simulink model "Cruise_MPC_Adaptive"  (R2018a)
settings: Solver=VariableStepAuto  StartTime=0.0  StopTime=inf  FixedStep=0.01  RelTol=1e-3  EnableMultiTasking=on
PreLoadFcn:
  | sampleTime = 0.05;
  | 
  | % Vehicle Parameters
  | R = 0.1;
  | L = 0.5;
undefined symbols (not defined in the file): C1, C2, cBW, d, Discrete, dw, I, Iw, md, Time, Waypoint
libraries: mobileRoboticsLib x2, cstblocks x2, mpclib x1, ctrlSharedLib x1, dspsrcs4 x1
settings Model: SimulationMode=accelerator  EnablePacing=on  Creator=scastro  LastModifiedBy=shravan
settings DataIOCC: LimitDataPoints=on
settings OptimizationCC: EfficientMapNaN2IntZero=off  LifeSpan=inf
settings DebuggingCC: AllowSymbolicDim=off  SFUnexpectedBacktrackingDiag=warning  SFNoUnconditionalDefaultTransitionDiag=warning  SFExecutionAtInitializationDiag=none
settings HardwareCC: TargetBitPerLong=64  TargetBitPerPointer=64  TargetBitPerSizeT=64  TargetBitPerPtrDiffT=64  TargetLongLongMode=on  TargetIntDivRoundTo=Zero  TargetEndianess=LittleEndian  TargetWordSize=64  TargetHWDeviceType=MATLAB Host  ProdEqTarget=off
settings CodeAppCC: MaxIdLength=128
settings GRTTargetCC: TargetLangStandard=C89/C90 (ANSI)  CombineOutputUpdateFcns=off  GRTInterface=on
settings ConfigComp: CovMetricSettings=dw  CovHtmlReporting=on  CovSaveCumulativeToWorkspaceVar=on  CovSaveSingleToWorkspaceVar=on  CovExternalEMLEnable=off  CovSFcnEnable=off
settings SimscapeCC: SimscapeNominalValues="[{\"value\":\"10\",\"unit\":\"V\"},{\"value\":\"1\",\"unit\":\"A\"},{\"value\":\"10\",\"unit\":\"N*m\"},{\"value\":\"10\",\"unit\":\"bar\"},{\"value\":\"100\",\"unit\":\"kJ/kg\"},{\"value\":\"1\",\"unit\":\"kW\"},{\"value\":\"300\",\"unit\":\"K\"},{\"value\":\"100\",\"unit\":\"cm^3/s\"},{\"value\":\"1\",\"unit\":\"kN\"},{\"value\":\"1\",\"unit\":\"g/cm^3\"},{\"value\":\"1\",\"unit\":\"l\"},{\"value\":\"1\",\"unit\":\"cm^2\"},{\"value\":\"60\",\"unit\":\"Hz\"}]"  SimscapeLogType=all  SimscapeLogDataHistory=10000
settings ConfigurationSet: Description=SimMechanics 2G
settings ExplorerConfigSet: InternalSimMechanicsExplorerSettings="<ExplorerConfiguration><canonicalview>default</canonicalview><AnimationSetting><BasePlaybackSpeed>1.0</BasePlaybackSpeed><PlaybackSpeedFactor>1.0</PlaybackSpeedFactor></AnimationSetting><TilePanel><TileInfo><Tiles Columns=\"1\" Count=\"1\" Rows=\"1\"><Column Weight=\"1\"/><Row Weight=\"1\"/><Tile Height=\"1\" Width=\"1\" X=\"0\" Y=\"0\"/></Tiles></TileInfo><SceneInfo><SceneViewer><BGColor><R>0.60000002384185791</R><G>0.60000002384185791</G><B>0.60000002384185791</B></BGColor><Camera><DoPerspective>off</DoPerspective><Position><X>-1.70656042355848525</X><Y>-0.974920623359631922</Y><Z>4.72930454537082046</Z></Position><Center><X>0.552860638431633689</X><Y>1.42025063411503494</Y><Z>1.4843509506914252</Z></Center><Up><X>0.664249622453917166</X><Y>0.300615402055903091</Y><Z>0.684399604848363485</Z></Up><ViewLimDist>1</ViewLimDist><YLim>2.77881717169207398</YLim><XLim>3.55928742670435394</XLim></Camera></SceneViewer></SceneInfo></TilePanel><MechEditorPanel><Cameras/><GfxPanelCameraMap/><VideoCreator><PlaybackSpeedRatio>1.0</PlaybackSpeedRatio><FrameRate>30</FrameRate><VideoFormat>Motion JPEG AVI</VideoFormat><FrameSize>auto</FrameSize></VideoCreator></MechEditorPanel></ExplorerConfiguration>"

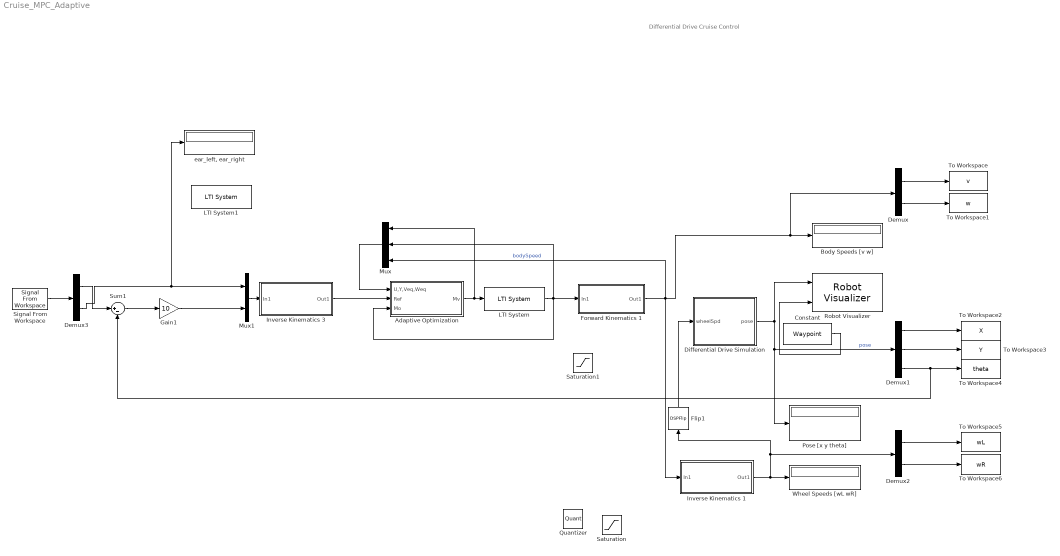
== system Cruise_MPC_Adaptive ==
  note: Differential Drive Cruise Control
  "Adaptive Optimization " : Subsystem
  Body Speeds [v w] : Display
  Constant : Constant  Value=Waypoint  SampleTime=sampleTime
  Demux : Demux  Outputs=2
  Demux1 : Demux  Outputs=3
  Demux2 : Demux  Outputs=2
  Demux3 : Demux  Outputs=2
  Differential Drive Simulation : Subsystem  AncestorBlock=mobileRoboticsLib/Kinematic Models/Differential Drive/Differential Drive Simulation  OverrideUsingVariant=mode==2  mask(Differential Drive Simulation){wheelRadius=R, wheelBase=L, initX=C1, initY=C2, initAngle=0, Ts=0.001}
      mask prompts: wheelRadius "Wheel Radius [m]"; wheelBase "Wheelbase [m]"; initX "Initial X Position [m]"; initY "Initial Y Position [m]"; initAngle "Initial Angle [rad]"; Ts "Sample Time"
      mask help:
      | Simulates the kinematics of a differential drive vehicle from a specified initial pose.
      |
      | Input: Left and right wheel speeds [wL; wR], in rad/s
      |
      | Output: Pose [x; y; theta], in m, m, and rad
      |
      | Set the Sample Time parameter to 0 for continuous-time simulation, or a positive number for discrete-time simulation.
      mask Help: web('matlab:edit mrsDocDifferentialDrive')
      mask Callback Ts:
      | Ts = evalin('base',get_param(gcb,'Ts'));
      | blk = [gcb '/Generic Robot Simulation/Velocity Integrator'];
      | if Ts > 0
      |     set_param(blk,'OverrideUsingVariant','mode==2');
      | else
      |     set_param(blk,'OverrideUsingVariant','mode==1');
      | end
  Flip1 : DSPFlip
  Forward Kinematics 1 : Subsystem
  Gain1 : Gain  Gain=10
  Inverse Kinematics 1 : Subsystem
  Inverse Kinematics 3 : Subsystem
  LTI System : cstblocks/LTI System  sys=Plant  IC=[0 0 0 0]
  LTI System1 : cstblocks/LTI System  sys=Controller  IC=[]
  Mux : Mux  Inputs=3
  Mux1 : Mux  Inputs=2
  Pose [x y theta] : Display
  Quantizer : Quantizer
  Robot Visualizer : mobileRoboticsLib/Environments/Robot Visualizer  Priority=99  robotRadius=1  showTrajectory=on  hasWaypoints=on  hasLidar=off  sensorOffset=[ 0 0 ]  scanAngles=[-pi/4,0,pi/4]  hasObjDetector=off  objDetectorOffset=[ 0, 0 ]  objDetectorAngle=0  objDetectorFOV=pi/4  objDetectorMaxRange=5  objectColors=[ 1, 0, 0; 0, 1, 0; 0, 0, 1 ]  objectMarkers='s'
      settings: SourceProductName=Mobile Robotics Simulation Library
  Saturation : Saturate
  Saturation1 : Saturate  UpperLimit=12  LowerLimit=0
  Signal From Workspace : dspsrcs4/Signal From Workspace  X=Cruise  Ts=cBW  nsamps=1  OutputAfterFinalValue=Holding final value  ignoreOrWarnInputAndFrameLengths=off  OutputFrames=off
  Sum1 : Sum  Inputs=|+-
  To Workspace : ToWorkspace  VariableName=v  SampleTime=-1
  To Workspace1 : ToWorkspace  VariableName=w  SampleTime=-1
  To Workspace2 : ToWorkspace  VariableName=X  SampleTime=sampleTime
  To Workspace3 : ToWorkspace  VariableName=Y  SampleTime=-1
  To Workspace4 : ToWorkspace  VariableName=theta  SampleTime=-1
  To Workspace5 : ToWorkspace  VariableName=wL  SampleTime=-1
  To Workspace6 : ToWorkspace  VariableName=wR  SampleTime=-1
  Wheel Speeds [wL wR] : Display
  "ear_left, ear_right " : Display
  wires:
  Differential Drive Simulation/1(pose) -> Demux1/1, Pose [x y theta]/1, Robot Visualizer/1  "pose"
  Forward Kinematics 1/1(Out1) -> Mux/3, Inverse Kinematics 1/1(In1), Demux/1, Body Speeds [v w]/1  "bodySpeed"
  Demux/1 -> To Workspace/1
  Demux/2 -> To Workspace1/1
  Demux1/1 -> To Workspace2/1
  Demux1/2 -> To Workspace3/1
  Demux2/1 -> To Workspace5/1
  Demux2/2 -> To Workspace6/1
  Constant/1 -> Robot Visualizer/2
  Inverse Kinematics 1/1(Out1) -> Demux2/1, Flip1/1, Wheel Speeds [wL wR]/1
  Signal From Workspace/1 -> Demux3/1
  Demux3/2 -> "ear_left, ear_right "/1, Mux1/1
  Demux3/1 -> Sum1/1
  Mux1/1 -> Inverse Kinematics 3/1(In1)
  Sum1/1 -> Gain1/1
  Gain1/1 -> Mux1/2
  Demux1/3 -> Sum1/2, To Workspace4/1
  LTI System/1 -> "Adaptive Optimization "/3(Mo), Mux/2, Forward Kinematics 1/1(In1)
  Flip1/1 -> Differential Drive Simulation/1(wheelSpd)
  "Adaptive Optimization "/1(Mv) -> Mux/1, LTI System/1
  Inverse Kinematics 3/1(Out1) -> "Adaptive Optimization "/2(Ref)
  Mux/1 -> "Adaptive Optimization "/1(U,Y,Veq,Weq)

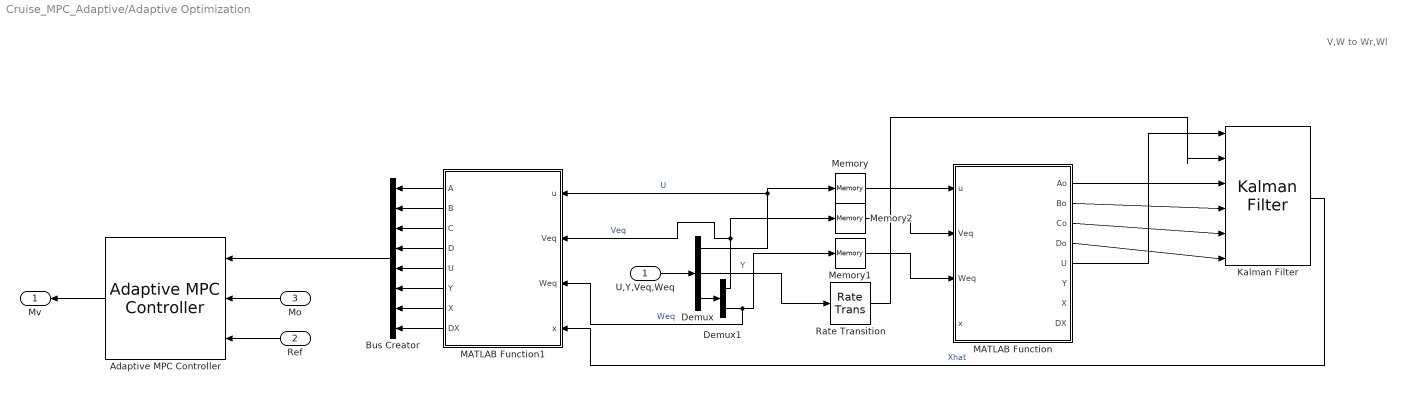
== system Cruise_MPC_Adaptive/Adaptive Optimization  ==
  note: V,W to Wr,Wl
  U,Y,Veq,Weq : Inport
  Ref : Inport  Port=2
  Mo : Inport  Port=3
  Adaptive MPC Controller : mpclib/Adaptive MPC Controller  SCDEnableBlockLinearizationSpecification=on  mpcobj=mpc1  updateMPCinCallerWorkspace=on  md_inport=off  mv_inport=off  cost_outport=off  return_sequence=off  return_qpstatus=off  return_state=off  state_inport=off  isltv_plant=off  lims_inport=off  cc_inport=off  ywt_inport=off  uwt_inport=off  duwt_inport=off  rhoeps_inport=off  uref_inport=off  BlockDataType=double  SampleTimeInherited=off  switch_inport=off
      settings: SourceProductName=Model Predictive Control Toolbox
  Bus Creator : BusCreator  Inputs=8
  Demux : Demux  Outputs=3
  Demux1 : Demux  Outputs=2
  Kalman Filter : ctrlSharedLib/Kalman Filter  TimeDomain=Discrete-Time  UseCurrentEstimator=on  ModelSource=Input port  ModelSourceVariable=Plant  A=0.95  B=1  C=1  D=0  NumberOfStates=4  NumberOfInputs=2  NumberOfOutputs=2  InitialEstimateSource=Dialog  X0=0  P0=0.1  UseK=off  UseGH=off  NumberOfProcessNoiseInputs=1  G=1  TimeInvariantG=on  H=0  TimeInvariantH=on  Q=diag([100 100 100 100])  TimeInvariantQ=on  R=diag([0.0001 0.0001])  TimeInvariantR=on  N=0  TimeInvariantN=on  AddInputPort=on  AddEnablePort=off  OutputEstimatedY=off  OutputP=off  Ts=sampleTime
      settings: SourceProductBaseCode=CT
  MATLAB Function : MATLAB Function  TreatAsAtomicUnit=on  SystemSampleTime=sampleTime
  MATLAB Function1 : MATLAB Function  TreatAsAtomicUnit=on  SystemSampleTime=sampleTime
  Memory : Memory
  Memory1 : Memory
  Memory2 : Memory
  Rate Transition : RateTransition  OutPortSampleTime=sampleTime
  Mv : Outport
  wires:
  U,Y,Veq,Weq/1 -> Demux/1
  Memory/1 -> MATLAB Function/1(u)
  Demux/1 -> Memory/1, MATLAB Function1/1(u)  "U"
  Memory2/1 -> MATLAB Function/2(Veq)
  Memory1/1 -> MATLAB Function/3(Weq)
  MATLAB Function/1(Ao) -> Kalman Filter/3
  MATLAB Function/2(Bo) -> Kalman Filter/4
  MATLAB Function/3(Co) -> Kalman Filter/5
  MATLAB Function/4(Do) -> Kalman Filter/6
  MATLAB Function/5(U) -> Kalman Filter/1
  Demux/2 -> Rate Transition/1  "Y"
  Rate Transition/1 -> Kalman Filter/2
  Kalman Filter/1 -> MATLAB Function1/4(x)  "Xhat"
  MATLAB Function1/1(A) -> Bus Creator/1
  MATLAB Function1/2(B) -> Bus Creator/2
  MATLAB Function1/3(C) -> Bus Creator/3
  MATLAB Function1/4(D) -> Bus Creator/4
  MATLAB Function1/5(U) -> Bus Creator/5
  MATLAB Function1/6(Y) -> Bus Creator/6
  MATLAB Function1/7(X) -> Bus Creator/7
  MATLAB Function1/8(DX) -> Bus Creator/8
  Bus Creator/1 -> Adaptive MPC Controller/1
  Mo/1 -> Adaptive MPC Controller/2
  Ref/1 -> Adaptive MPC Controller/3
  Adaptive MPC Controller/1 -> Mv/1
  Demux/3 -> Demux1/1
  Demux1/1 -> MATLAB Function1/2(Veq), Memory2/1  "Veq"
  Demux1/2 -> MATLAB Function1/3(Weq), Memory1/1  "Weq"

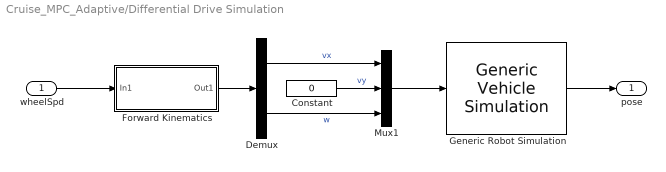
== system Cruise_MPC_Adaptive/Differential Drive Simulation ==
  wheelSpd : Inport
  Constant : Constant  Value=0
  Demux : Demux  Outputs=2
  "Forward Kinematics " : Subsystem
  Generic Robot Simulation : mobileRoboticsLib/Utilities/Generic Vehicle Simulation  initX=initX  initY=initY  initAngle=initAngle  Ts=Ts
      link override Velocity Integrator: OverrideUsingVariant=mode==2
      settings: SourceProductName=Mobile Robotics Simulation Toolbox
  Mux1 : Mux  Inputs=3
  pose : Outport
  wires:
  Generic Robot Simulation/1 -> pose/1
  "Forward Kinematics "/1(Out1) -> Demux/1
  wheelSpd/1 -> "Forward Kinematics "/1(In1)
  Constant/1 -> Mux1/2  "vy"
  Demux/2 -> Mux1/3  "w"
  Demux/1 -> Mux1/1  "vx"
  Mux1/1 -> Generic Robot Simulation/1

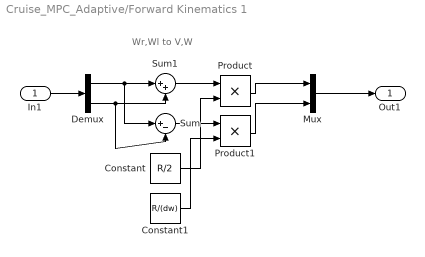
== system Cruise_MPC_Adaptive/Forward Kinematics 1 ==
  note: Wr,Wl to V,W
  In1 : Inport
  Constant : Constant  Value=R/2
  Constant1 : Constant  Value=R/(dw)
  Demux : Demux  Outputs=2
  Mux : Mux  Inputs=2
  Product : Product
  Product1 : Product
  Sum : Sum  Inputs=|+-
  Sum1 : Sum  Inputs=|++
  Out1 : Outport
  wires:
  In1/1 -> Demux/1
  Product1/1 -> Mux/2
  Mux/1 -> Out1/1
  Product/1 -> Mux/1
  Demux/1 -> Sum/1, Sum1/1
  Demux/2 -> Sum/2, Sum1/2
  Sum1/1 -> Product/1
  Constant/1 -> Product/2
  Sum/1 -> Product1/1
  Constant1/1 -> Product1/2

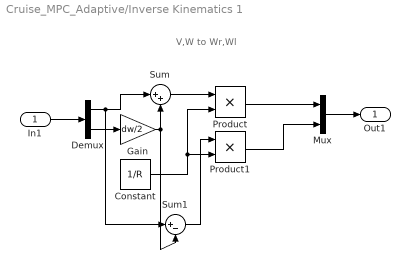
== system Cruise_MPC_Adaptive/Inverse Kinematics 1 ==
  note: V,W to Wr,Wl
  In1 : Inport
  Constant : Constant  Value=1/R
  Demux : Demux  Outputs=2
  Gain : Gain  Gain=dw/2
  Mux : Mux  Inputs=2
  Product : Product
  Product1 : Product
  Sum : Sum  Inputs=|++
  Sum1 : Sum  Inputs=|+-
  Out1 : Outport
  wires:
  Gain/1 -> Sum/2, Sum1/2
  Product1/1 -> Mux/2
  Product/1 -> Mux/1
  Sum1/1 -> Product1/1
  Constant/1 -> Product/2, Product1/2
  Sum/1 -> Product/1
  Demux/1 -> Sum/1, Sum1/1
  Demux/2 -> Gain/1
  In1/1 -> Demux/1
  Mux/1 -> Out1/1

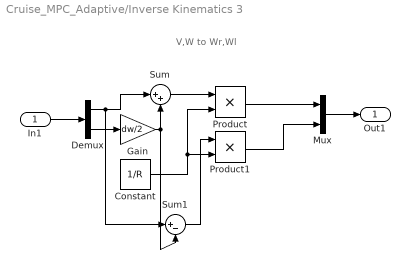
== system Cruise_MPC_Adaptive/Inverse Kinematics 3 ==
  note: V,W to Wr,Wl
  In1 : Inport
  Constant : Constant  Value=1/R
  Demux : Demux  Outputs=2
  Gain : Gain  Gain=dw/2
  Mux : Mux  Inputs=2
  Product : Product
  Product1 : Product
  Sum : Sum  Inputs=|++
  Sum1 : Sum  Inputs=|+-
  Out1 : Outport
  wires:
  Gain/1 -> Sum/2, Sum1/2
  Product1/1 -> Mux/2
  Product/1 -> Mux/1
  Sum1/1 -> Product1/1
  Constant/1 -> Product/2, Product1/2
  Sum/1 -> Product/1
  Demux/1 -> Sum/1, Sum1/1
  Demux/2 -> Gain/1
  In1/1 -> Demux/1
  Mux/1 -> Out1/1

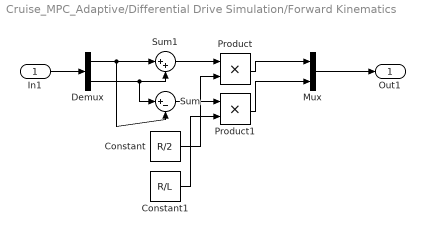
== system Cruise_MPC_Adaptive/Differential Drive Simulation/Forward Kinematics  ==
  In1 : Inport
  Constant : Constant  Value=R/2
  Constant1 : Constant  Value=R/L
  Demux : Demux  Outputs=2
  Mux : Mux  Inputs=2
  Product : Product
  Product1 : Product
  Sum : Sum  Inputs=|+-
  Sum1 : Sum  Inputs=|++
  Out1 : Outport
  wires:
  In1/1 -> Demux/1
  Product1/1 -> Mux/2
  Mux/1 -> Out1/1
  Product/1 -> Mux/1
  Demux/1 -> Sum/2, Sum1/1
  Demux/2 -> Sum/1, Sum1/2
  Sum1/1 -> Product/1
  Constant/1 -> Product/2
  Sum/1 -> Product1/1
  Constant1/1 -> Product1/2

== matlab function Cruise_MPC_Adaptive/Adaptive Optimization /MATLAB Function ==
  data: u input size=[2,1]; Veq input size=[1,1]; Weq input size=[1,1]; Ao output size=[4,4]; x input size=[4,1]; Bo output size=[4,2]; Co output size=[2,4]; Do output size=[2,2]; U output size=[2,1]; Y output size=[2,1]; X output size=[4,1]; DX output size=[4,1]; sampleTime parameter size=[1,1]; d parameter size=[1,1]; dw parameter size=[1,1]; Iw parameter size=[1,1]; I parameter size=[1,1]; md parameter size=1,1; R parameter size=1,1; L parameter size=1,1
function [Ao,Bo,Co,Do,U,Y,X,DX] = fcn(u,Veq,Weq,x,sampleTime,d, dw, Iw, I, md, R, L)
% Sample time
Ts = sampleTime;

% Model Parameters
Kt = 0.0046; Kg = 50; Kb = Kt; Beta = 2.29e-06; La =1.729e-03; Ra = 5.51;
m = 3.4; mc = 2.76 + md; I = I ; Iw = Iw; L = L; d = d; dw = dw; 
A = m + 2*Iw/(R*R); B = I + dw*dw*Iw/(2*R*R);

% Continuous-time model for Plant e_r, e_l to Wr,Wl
Ac = [-2*Beta*Kg*Kg/(A*R*R)  2*mc*d*Weq/A   (Kt*Kg/(R*A))  (Kt*Kg/(A*R));
      -mc*d*Weq/B  (-mc*d*Veq/B)-(Beta*dw*dw*Kg*Kg/(2*R*R*B)) dw*Kt*Kg/(2*R*B) -dw*Kt*Kg/(2*B*R) ;
     -Kb*Kg/(La*R)   -Kb*Kg*dw/(2*La*R)  -Ra/La      0 ;
     -Kb*Kg/(La*R)    Kb*Kg*dw/(2*La*R)    0       -Ra/La ];
Bc = [0 0; 0 0; 1/La 0; 0 1/La]; Cc =  [1/R dw/(2*R); 1/R -dw/(2*R)]*[1 0 0 0; 0 1 0 0]; Dc = [0 0;0 0];


% Discretize the continuous-time model using zero-order hold 
% on the inputs and a sample time of Ts seconds
nx = size(Ac,1);
nu = size(Bc,2);
M = expm([[Ac Bc]*Ts; zeros(nu,nx+nu)]);
Ao = M(1:nx,1:nx);
Bo = M(1:nx,nx+1:nx+nu);
Co = Cc;
Do = Dc;

% Nominal conditions for discrete-time plant
X = x;
U = u;
Y = Co*x + Do*u;
DX = Ao*x+Bo*u-x;

== matlab function Cruise_MPC_Adaptive/Adaptive Optimization /MATLAB Function1 ==
  data: u input size=[2,1]; Veq input size=[1,1]; Weq input size=[1,1]; A output size=[4,4]; x input size=[4,1]; B output size=[4,2]; C output size=[2,4]; D output size=[2,2]; U output size=[2,1]; Y output size=[2,1]; X output size=[4,1]; DX output size=[4,1]; sampleTime parameter size=[1,1]; d parameter size=[1,1]; dw parameter size=[1,1]; Iw parameter size=[1,1]; I parameter size=[1,1]; md parameter size=1,1; R parameter size=1,1; L parameter size=1,1
function [A,B,C,D,U,Y,X,DX] = fcn(u,Veq,Weq,x,sampleTime,d, dw, Iw, I, md, R, L)
% Sample time
Ts = sampleTime;

% Model Parameters
Kt = 0.0046; Kg = 50; Kb = Kt; Beta = 2.29e-06; La =1.729e-03; Ra = 5.51;
m = 3.4; mc = 2.76 + md; I = I ; Iw = Iw; L = L; d = d; dw = dw; 
Ao = m + 2*Iw/(R*R); Bo = I + dw*dw*Iw/(2*R*R);

% Continuous-time model for Plant e_r, e_l to Wr,Wl
Ac = [-2*Beta*Kg*Kg/(Ao*R*R)  2*mc*d*Weq/Ao   (Kt*Kg/(R*Ao))  (Kt*Kg/(Ao*R));
      -mc*d*Weq/Bo  (-mc*d*Veq/Bo)-(Beta*dw*dw*Kg*Kg/(2*R*R*Bo)) dw*Kt*Kg/(2*R*Bo) -dw*Kt*Kg/(2*Bo*R) ;
     -Kb*Kg/(La*R)   -Kb*Kg*dw/(2*La*R)  -Ra/La      0 ;
     -Kb*Kg/(La*R)    Kb*Kg*dw/(2*La*R)    0       -Ra/La ];
Bc = [0 0; 0 0; 1/La 0; 0 1/La]; Cc =  [1/R dw/(2*R); 1/R -dw/(2*R)]*[1 0 0 0; 0 1 0 0]; Dc = [0 0;0 0];


% Discretize the continuous-time model using zero-order hold 
% on the inputs and a sample time of Ts seconds
nx = size(Ac,1);
nu = size(Bc,2);
M = expm([[Ac Bc]*Ts; zeros(nu,nx+nu)]);
A = M(1:nx,1:nx);
B = M(1:nx,nx+1:nx+nu);
C = Cc;
D = Dc;

% Nominal conditions for discrete-time plant
X = x;
U = u;
Y = C*x + D*u;
DX = A*x+B*u-x;
